simulink model "aeroblk_HL20_DG"  (Simulink 6.0)
settings: Solver=ode45  StartTime=0.0  StopTime=100  RelTol=1e-3
PreLoadFcn:
  | aeroblk_init_HL20
values from neighbouring files (symbols this model uses):
  Act2Aero = 0.5*[1 -1 0 0 0 0 0;1 1 0 0 0 0 0 ;0 0 0 0 0 0 2;0 0 1 1 0 0 0; 0 0 0 0 1 1 0;0 0 1 -1 1 -1 0;]    [aeroblk_init_HL20.m]
  Aero2Act = pinv(Act2Aero)    [aeroblk_init_HL20.m]
  Aimpoint = 12071.9115088    [aeroblk_HL20_glideslope.mat]    (also in aeroblk_init_HL20.m = 0)
  alpha0 = 0.114253174362    [aeroblk_HL20_glideslope.mat]
  hglide = [0 2.62038896415 5.2407779283 7.86116689246 10.4815558566 13.1019448208 15.7223337849 18.3427227491 20.9631117132 23.5835006774 26.2038896415 28.8242786057 ... (301 elements, 1x301)]    [aeroblk_HL20_glideslope.mat]
  qbar0 = 10722.8924586    [aeroblk_HL20_autopilot_gains.mat]
  U_trim_matrix = [-23.7683817467 -4.33440943636 4.43733647183 -22.1955716586 4.52075664841 21.6532360323 -20.4783849922 6.34956743865 19.7065472455 -22.2662158495 5.88613316784 30.8883374276 ... (120 elements, 3x8x5)]    [aeroblk_HL20_autopilot_gains.mat]
  Xglide = [0 50 100 150 200 250 300 350 400 450 500 550 ... (301 elements, 1x301)]    [aeroblk_HL20_glideslope.mat]
undefined symbols (not defined in the file or in its folder): ft, m, s
libraries: aerolibconvert x13, simulink x5, simulink3 x5, dnglibv1 x5, aeroblk_lib_HL20 x3, aerolibactuator x1
settings Model: Creator=sgage  ModifiedByFormat=rhyde  LastModifiedBy=rhyde  ModifiedComment=rhyde -- Wed Mar 13 13:42:21 2002 -- Version 1.0  ModifiedHistory=A.N.Other -- Wed Mar 13 13:42:21 2002 -- Version 1.0  ExtModeAutoUpdateStatusClock=off
settings DataIOCC: SignalLoggingName=sigsOut
settings OptimizationCC: BooleanDataType=off  InlineParams=on
settings DebuggingCC: CheckExecutionContextPreStartOutputMsg=on  CheckExecutionContextRuntimeOutputMsg=on  SolverPrmCheckMsg=none
settings HardwareCC: TargetUnknown=on
settings GRTTargetCC: LifeSpan=inf
settings SFSimCC: SFSimApplyToAllLibs=on  SFSimBuildMode=Incremental

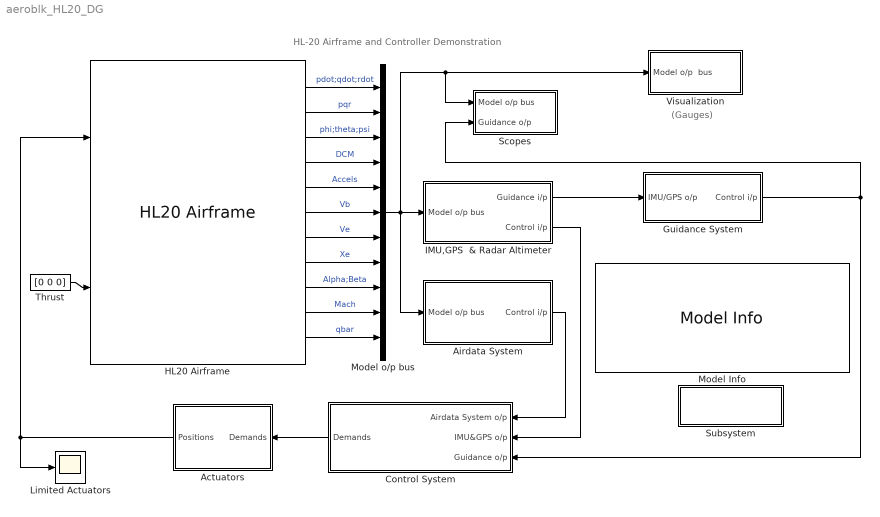
== system aeroblk_HL20_DG ==
  note: HL-20 Airframe and Controller Demonstration
  note: (Gauges)
  Actuators : Subsystem  Orientation=left  PropExecContextAcrossSSBoundary=on
  Airdata System : Subsystem  PropExecContextAcrossSSBoundary=on
  Control System : Subsystem  Orientation=left  PropExecContextAcrossSSBoundary=on
  Guidance System : Subsystem  PropExecContextAcrossSSBoundary=on
  HL20 Airframe : aeroblk_lib_HL20/HL20 Airframe
  IMU,GPS  & Radar Altimeter : Subsystem  PropExecContextAcrossSSBoundary=on
  Limited Actuators : Scope
      settings: YMin=-60  YMax=60  SaveName=ScopeData2
  Model o/p bus : BusCreator  DialogController=Simulink.DDGSource_Bus  Inputs=11
  Model Info : simulink/Model-Wide Utilities/Model Info  InitialBlockCM=None  BlockCM=None  Frame=on  DisplayStringWithTags=|  HorizontalTextAlignment=Center  LeftAlignmentValue=0.5  SourceBlockDiagram=aeroblk_HL20_DG  TagMaxNumber=20
      | HL20 version %<ModelVersion>
      | Modified on %<LastModificationDate>
      | based on 
      | Jackson E. B., Cruz C. L., 
      | "Preliminary Subsonic Aerodynamic Model for
      | Simulation Studies of the HL-20 Lifting Body", 
      | NASA TM4302, August 1992.%<Description>
  Scopes : Subsystem  PropExecContextAcrossSSBoundary=on
  Subsystem : Subsystem  PropExecContextAcrossSSBoundary=on
      settings: OpenFcn=aeroblk_lib_HL20
      mask Display: disp('Open HL20 Library')
  Thrust : Constant  Value=[0 0 0]
  Visualization : Subsystem  PropExecContextAcrossSSBoundary=on
  wires:
  Thrust/1 -> HL20 Airframe/2
  Actuators/1(Positions) -> Limited Actuators/1, HL20 Airframe/1
  Guidance System/1(Control i/p) -> Control System/3(Guidance o/p), Scopes/2(Guidance o/p)
  Control System/1(Demands) -> Actuators/1(Demands)
  HL20 Airframe/1 -> Model o/p bus/1  "pdot;qdot;rdot"
  HL20 Airframe/2 -> Model o/p bus/2  "pqr"
  HL20 Airframe/3 -> Model o/p bus/3  "phi;theta;psi"
  HL20 Airframe/4 -> Model o/p bus/4  "DCM"
  HL20 Airframe/5 -> Model o/p bus/5  "Accels"
  HL20 Airframe/6 -> Model o/p bus/6  "Vb"
  HL20 Airframe/7 -> Model o/p bus/7  "Ve"
  HL20 Airframe/8 -> Model o/p bus/8  "Xe"
  HL20 Airframe/9 -> Model o/p bus/9  "Alpha;Beta"
  HL20 Airframe/10 -> Model o/p bus/10  "Mach"
  HL20 Airframe/11 -> Model o/p bus/11  "qbar"
  Model o/p bus/1 -> Airdata System/1(Model o/p bus), IMU,GPS  & Radar Altimeter/1(Model o/p bus), Visualization/1(Model o/p  bus), Scopes/1(Model o/p bus)
  IMU,GPS  & Radar Altimeter/2(Control i/p) -> Control System/2(IMU&GPS o/p)
  Airdata System/1(Control i/p) -> Control System/1(Airdata System o/p)
  IMU,GPS  & Radar Altimeter/1(Guidance i/p) -> Guidance System/1(IMU/GPS o/p)

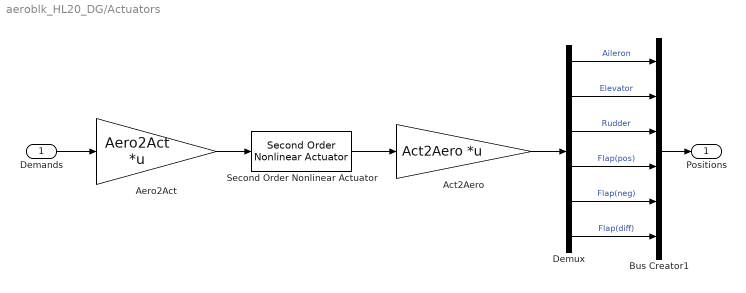
== system aeroblk_HL20_DG/Actuators ==
  Demands : Inport  LatchInput=off
  Act2Aero : Gain  Gain=Act2Aero  Multiplication=Matrix(K*u)  SaturateOnIntegerOverflow=on
  Aero2Act : Gain  Gain=Aero2Act  Multiplication=Matrix(K*u)  SaturateOnIntegerOverflow=on
  Bus Creator1 : BusCreator  DialogController=Simulink.DDGSource_Bus  Inputs=6
  Demux : Demux  Outputs=6
  Second Order Nonlinear Actuator : aerolibactuator/Second Order Nonlinear Actuator  wn_fin=wn_act  z_fin=z_act  fin_max=max_lim  fin_min=min_lim  fin_maxrate=inf  fin_act_0=0
  Positions : Outport
  wires:
  Demux/1 -> Bus Creator1/1  "Aileron"
  Demux/2 -> Bus Creator1/2  "Elevator"
  Demux/3 -> Bus Creator1/3  "Rudder"
  Demux/4 -> Bus Creator1/4  "Flap(pos)"
  Demux/5 -> Bus Creator1/5  "Flap(neg)"
  Demux/6 -> Bus Creator1/6  "Flap(diff)"
  Bus Creator1/1 -> Positions/1
  Second Order Nonlinear Actuator/1 -> Act2Aero/1
  Aero2Act/1 -> Second Order Nonlinear Actuator/1
  Act2Aero/1 -> Demux/1
  Demands/1 -> Aero2Act/1

== system aeroblk_HL20_DG/Airdata System ==
  Model o/p bus : Inport  LatchInput=off
  Bus Selector : BusSelector  DialogController=Simulink.DDGSource_Bus  OutputSignals=Alpha;Beta,qbar
  Mux : Mux  Inputs=[2,1]
  Control i/p : Outport
  wires:
  Model o/p bus/1 -> Bus Selector/1
  Bus Selector/1 -> Mux/1  "<Alpha;Beta>"
  Bus Selector/2 -> Mux/2  "<qbar>"
  Mux/1 -> Control i/p/1

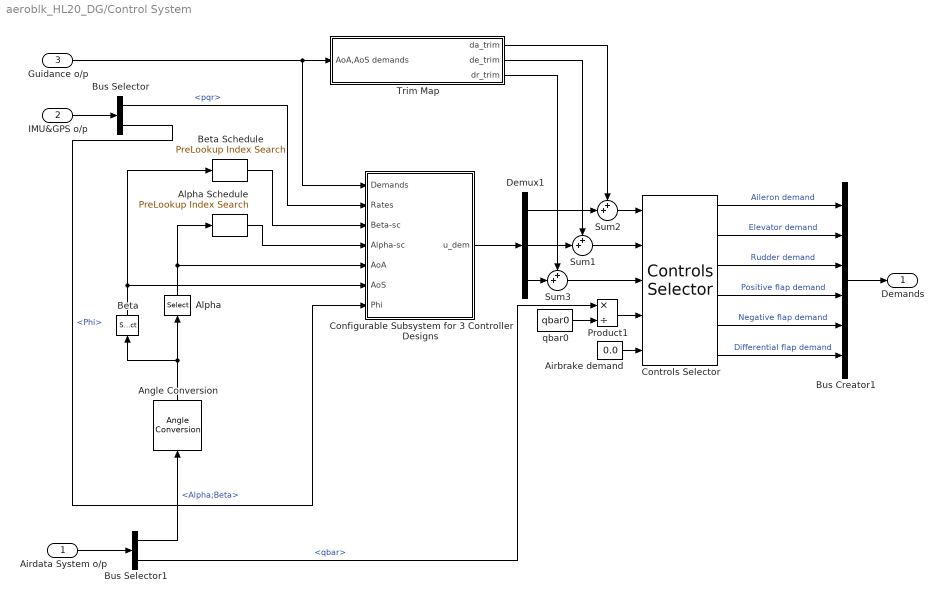
== system aeroblk_HL20_DG/Control System ==
  Airdata System o/p : Inport  LatchInput=off
  IMU&GPS o/p : Inport  Port=2  LatchInput=off
  Guidance o/p : Inport  Port=3  LatchInput=off
  Airbrake demand : Constant  Value=0.0
  Alpha : Selector  Orientation=up  InputPortWidth=2
  Alpha Schedule : simulink/Lookup Tables/PreLookup Index Search  bpData=a_vec  searchMode=Binary Search  cacheBpFlag=off  outputFlag=off  extrapMode=Linear Extrapolation  rangeErrorMode=None
  Angle Conversion : aerolibconvert/Angle Conversion  Orientation=up  IU=rad  OU=deg
  Beta : Selector  Orientation=up  Elements=2  InputPortWidth=2
  Beta Schedule : simulink/Lookup Tables/PreLookup Index Search  bpData=a_vec  searchMode=Binary Search  cacheBpFlag=off  outputFlag=off  extrapMode=Linear Extrapolation  rangeErrorMode=None
  Bus Creator1 : BusCreator  DialogController=Simulink.DDGSource_Bus  Inputs=6
  Bus Selector : BusSelector  DialogController=Simulink.DDGSource_Bus  OutputSignals=pqr,Phi
  Bus Selector1 : BusSelector  DialogController=Simulink.DDGSource_Bus  OutputSignals=Alpha;Beta,qbar
  Configurable Subsystem for 3 Controller Designs : Subsystem  BlockChoice=Classical Controller  PropExecContextAcrossSSBoundary=on
      settings: AttributesFormatString=%<BlockChoice>  MemberBlocks=Classical Controller,H-infinity Controller [1 dimensional scheduling],H-infinity Controller [2 dimensional scheduling]
      settings: TemplateBlock=|
      | aeroblk_lib_HL20/Configurable Subsystem
      | for 3 Controller Designs
  Controls Selector : aeroblk_lib_HL20/Controls Selector  SimViewingDevice=off  DataTypeOverride=UseLocalSettings  MinMaxOverflowLogging=UseLocalSettings
      settings: Permissions=ReadWrite  RTWFcnNameOpts=Auto  RTWFileNameOpts=Auto
  Demux1 : Demux  Outputs=3
  Product1 : Product  Inputs=*/  SaturateOnIntegerOverflow=on  InputSameDT=on
  Sum1 : Sum  Inputs=++|  SaturateOnIntegerOverflow=on  InputSameDT=on
  Sum2 : Sum  Inputs=++|  SaturateOnIntegerOverflow=on  InputSameDT=on
  Sum3 : Sum  Inputs=++|  SaturateOnIntegerOverflow=on  InputSameDT=on
  Trim Map : Subsystem  PropExecContextAcrossSSBoundary=on
  qbar0 : Constant  Value=qbar0
  Demands : Outport
  wires:
  Bus Creator1/1 -> Demands/1
  Alpha Schedule/1 -> Configurable Subsystem for 3 Controller Designs/4(Alpha-sc)
  Beta Schedule/1 -> Configurable Subsystem for 3 Controller Designs/3(Beta-sc)
  Bus Selector/1 -> Configurable Subsystem for 3 Controller Designs/2(Rates)  "<pqr>"
  Guidance o/p/1 -> Trim Map/1(AoA,AoS demands), Configurable Subsystem for 3 Controller Designs/1(Demands)
  Alpha/1 -> Alpha Schedule/1, Configurable Subsystem for 3 Controller Designs/5(AoA)
  Angle Conversion/1 -> Beta/1, Alpha/1
  Controls Selector/1 -> Bus Creator1/1  "Aileron demand"
  Controls Selector/2 -> Bus Creator1/2  "Elevator demand"
  Controls Selector/3 -> Bus Creator1/3  "Rudder demand"
  Controls Selector/4 -> Bus Creator1/4  "Positive flap demand"
  Controls Selector/5 -> Bus Creator1/5  "Negative flap demand"
  Controls Selector/6 -> Bus Creator1/6  "Differential flap demand"
  Beta/1 -> Beta Schedule/1, Configurable Subsystem for 3 Controller Designs/6(AoS)
  Product1/1 -> Controls Selector/4
  qbar0/1 -> Product1/2
  Sum2/1 -> Controls Selector/1
  Trim Map/1(da_trim) -> Sum2/1
  Sum1/1 -> Controls Selector/2
  Sum3/1 -> Controls Selector/3
  Trim Map/2(de_trim) -> Sum1/1
  Trim Map/3(dr_trim) -> Sum3/1
  Demux1/2 -> Sum1/2
  Demux1/3 -> Sum3/2
  Demux1/1 -> Sum2/2
  Configurable Subsystem for 3 Controller Designs/1(u_dem) -> Demux1/1
  IMU&GPS o/p/1 -> Bus Selector/1
  Bus Selector/2 -> Configurable Subsystem for 3 Controller Designs/7(Phi)  "<Phi>"
  Airdata System o/p/1 -> Bus Selector1/1
  Bus Selector1/1 -> Angle Conversion/1  "<Alpha;Beta>"
  Bus Selector1/2 -> Product1/1  "<qbar>"
  Airbrake demand/1 -> Controls Selector/5

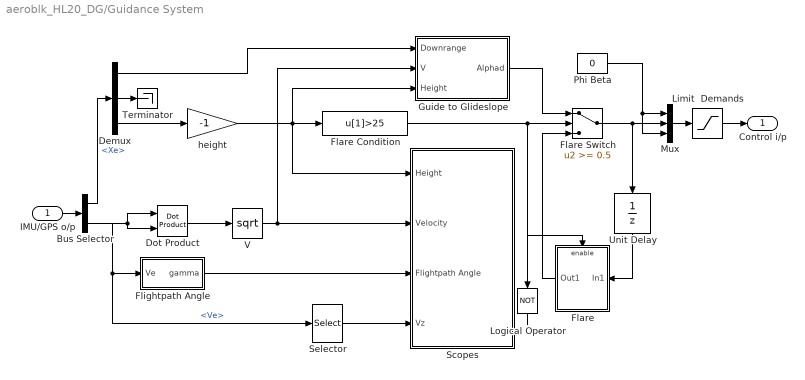
== system aeroblk_HL20_DG/Guidance System ==
  IMU/GPS o/p : Inport  LatchInput=off
  Bus Selector : BusSelector  DialogController=Simulink.DDGSource_Bus  OutputSignals=Xe,Ve
  Demux : Demux  Outputs=3
  Dot Product : simulink/Math Operations/Dot Product  OutDataType=sfix(16)  OutScaling=2^-10  DoSatur=on
  Flare : Subsystem  Orientation=left  TreatAsAtomicUnit=on  PropExecContextAcrossSSBoundary=on
  Flare Condition : Fcn  Expr=u[1]>25
  Flare Switch : Switch  Threshold=0.5  SaturateOnIntegerOverflow=on  InputSameDT=on
  Flightpath Angle : Subsystem  PropExecContextAcrossSSBoundary=on
  Guide to Glideslope : Subsystem  PropExecContextAcrossSSBoundary=on
  Limit  Demands : Saturate  UpperLimit=[20 25 5]  LowerLimit=[-20 -10 -5]
  Logical Operator : Logic  Orientation=down  Operator=NOT
  Mux : Mux  Inputs=3
  Phi Beta : Constant  Value=0
  Scopes : Subsystem  PropExecContextAcrossSSBoundary=on
  Selector : Selector  Elements=[3]  InputPortWidth=3
  Terminator : Terminator
  Unit Delay : UnitDelay  Orientation=down  SampleTime=0.1
  V : Math  Operator=sqrt  SaturateOnIntegerOverflow=on
  height : Gain  Gain=-1  SaturateOnIntegerOverflow=on
  Control i/p : Outport
  wires:
  Dot Product/1 -> V/1
  Unit Delay/1 -> Flare/1(In1)
  Logical Operator/1 -> Flare/Enable
  Demux/2 -> Terminator/1
  Guide to Glideslope/1(Alphad) -> Flare Switch/1
  Limit  Demands/1 -> Control i/p/1
  Flare/1(Out1) -> Flare Switch/3
  Flare Switch/1 -> Unit Delay/1, Mux/2
  Flare Condition/1 -> Logical Operator/1, Flare Switch/2
  Phi Beta/1 -> Mux/1, Mux/3
  Selector/1 -> Scopes/4(Vz)
  V/1 -> Scopes/2(Velocity), Guide to Glideslope/2(V)
  Mux/1 -> Limit  Demands/1
  height/1 -> Scopes/1(Height), Guide to Glideslope/3(Height), Flare Condition/1
  Demux/3 -> height/1
  Demux/1 -> Guide to Glideslope/1(Downrange)
  Bus Selector/1 -> Demux/1  "<Xe>"
  Flightpath Angle/1(gamma) -> Scopes/3(Flightpath Angle)
  Bus Selector/2 -> Flightpath Angle/1(Ve), Dot Product/2, Dot Product/1, Selector/1  "<Ve>"
  IMU/GPS o/p/1 -> Bus Selector/1

== system aeroblk_HL20_DG/IMU,GPS  & Radar Altimeter ==
  Model o/p bus : Inport  LatchInput=off
  Bus Creator : BusCreator  DialogController=Simulink.DDGSource_Bus  Inputs=7
  Bus Selector : BusSelector  DialogController=Simulink.DDGSource_Bus  OutputSignals=pqr,phi;theta;psi,DCM,Accels,Vb,Ve,Xe
  Mux : Mux  Inputs=[3,1]
  Select Phi : Selector  Elements=[1]  InputPortWidth=3
  Guidance i/p : Outport
  Control i/p : Outport  Port=2
  wires:
  Model o/p bus/1 -> Bus Selector/1
  Bus Selector/1 -> Bus Creator/1, Mux/1  "<pqr>"
  Bus Selector/2 -> Bus Creator/2, Select Phi/1  "<phi;theta;psi>"
  Bus Selector/3 -> Bus Creator/3  "<DCM>"
  Bus Selector/4 -> Bus Creator/4  "<Accels>"
  Bus Selector/5 -> Bus Creator/5  "<Vb>"
  Bus Selector/6 -> Bus Creator/6  "<Ve>"
  Bus Selector/7 -> Bus Creator/7  "<Xe>"
  Bus Creator/1 -> Guidance i/p/1
  Select Phi/1 -> Mux/2  "Phi"
  Mux/1 -> Control i/p/1

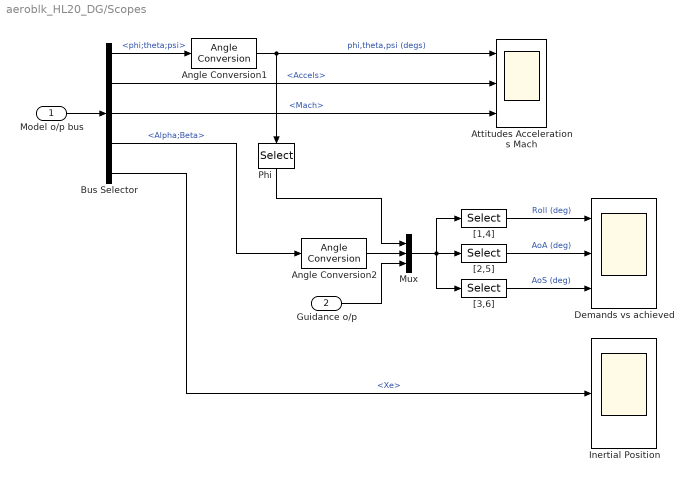
== system aeroblk_HL20_DG/Scopes ==
  Model o/p bus : Inport  LatchInput=off
  Guidance o/p : Inport  Port=2  LatchInput=off
  Angle Conversion1 : aerolibconvert/Angle Conversion  IU=rad  OU=deg
  Angle Conversion2 : aerolibconvert/Angle Conversion  IU=rad  OU=deg
  Attitudes Accelerations Mach : Scope  NumInputPorts=3
      settings: YMin=-11~-1.25~0.581  YMax=1~1.75~0.595  SaveName=ScopeData3  Decimation=5
  Bus Selector : BusSelector  DialogController=Simulink.DDGSource_Bus  OutputSignals=phi;theta;psi,Accels,Mach,Alpha;Beta,Xe
  Demands vs achieved : Scope  NumInputPorts=3
      settings: TimeRange=100  YMin=-0.6~2.5~-0.7  YMax=0.7~22.5~0.6  Decimation=5
  Inertial Position : Scope
      settings: TimeRange=100  YMin=-13000  YMax=1000  Decimation=5
  Mux : Mux  Inputs=[1,2,3]
  Phi : Selector  Orientation=down  InputPortWidth=3
  "[1,4]" : Selector  Elements=[1 4]  InputPortWidth=6
  "[2,5]" : Selector  Elements=[2 5]  InputPortWidth=6
  "[3,6]" : Selector  Elements=[3 6]  InputPortWidth=6
  wires:
  Model o/p bus/1 -> Bus Selector/1
  Bus Selector/1 -> Angle Conversion1/1  "<phi;theta;psi>"
  Bus Selector/2 -> Attitudes Accelerations Mach/2  "<Accels>"
  Bus Selector/3 -> Attitudes Accelerations Mach/3  "<Mach>"
  Phi/1 -> Mux/1
  Bus Selector/4 -> Angle Conversion2/1  "<Alpha;Beta>"
  Angle Conversion2/1 -> Mux/2
  Mux/1 -> "[1,4]"/1, "[2,5]"/1, "[3,6]"/1
  Guidance o/p/1 -> Mux/3
  "[1,4]"/1 -> Demands vs achieved/1  "Roll (deg)"
  "[2,5]"/1 -> Demands vs achieved/2  "AoA (deg)"
  "[3,6]"/1 -> Demands vs achieved/3  "AoS (deg)"
  Bus Selector/5 -> Inertial Position/1  "<Xe>"
  Angle Conversion1/1 -> Phi/1, Attitudes Accelerations Mach/1  "phi,theta,psi (degs)"

== system aeroblk_HL20_DG/Subsystem ==

== system aeroblk_HL20_DG/Visualization ==
  Model o/p  bus : Inport  LatchInput=off
  AirSpeed : dnglibv1/ActiveX Control  progid=air.airctrl.1  connect=input  input=airspeed  init=hActx.displaymode=4;  inblock=on  border=off  dialOut=0  updateParam=0
  Altimeter : dnglibv1/ActiveX Control  progid=air.airctrl.1  connect=input  input=altitude  init=hActx.displaymode=2;hActx.altthousandstyle=1;  inblock=on  border=off  dialOut=0  updateParam=0
  Artificial Horizon : dnglibv1/ActiveX Control  progid=air.airctrl.1  connect=input  input=ahroll, ahpitch  init=hActx.displaymode=6;  inblock=on  border=off  dialOut=0  updateParam=0
  Climb Rate : dnglibv1/ActiveX Control  progid=air.airctrl.1  connect=input  input=climbrate  init=hActx.displaymode=3;  inblock=on  border=off  dialOut=0  updateParam=0
  Extract Gauges : Subsystem  PropExecContextAcrossSSBoundary=on
  Heading Indicator : dnglibv1/ActiveX Control  progid=air.airctrl.1  connect=input  init=hActx.displaymode=1;  inblock=on  border=off  dialOut=0  updateParam=0
  wires:
  Model o/p  bus/1 -> Extract Gauges/1(Demands)
  Extract Gauges/1(Airspeed (kts)) -> AirSpeed/1
  Extract Gauges/5(Heading (deg)) -> Heading Indicator/1
  Extract Gauges/2(Height (ft)) -> Altimeter/1
  Extract Gauges/4(Climb Rate (ft/min)) -> Climb Rate/1
  Extract Gauges/3(Roll Flightpath (deg)) -> Artificial Horizon/1

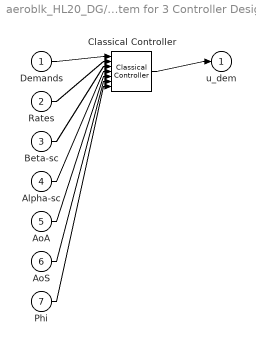
== system aeroblk_HL20_DG/Control System/Configurable Subsystem for 3 Controller Designs ==
  Demands : Inport  LatchInput=off
  Rates : Inport  Port=2  LatchInput=off
  Beta-sc : Inport  Port=3  LatchInput=off
  Alpha-sc : Inport  Port=4  LatchInput=off
  AoA : Inport  Port=5  LatchInput=off
  AoS : Inport  Port=6  LatchInput=off
  Phi : Inport  Port=7  LatchInput=off
  Classical Controller : aeroblk_lib_HL20/Classical Controller  SimViewingDevice=off  DataTypeOverride=UseLocalSettings  MinMaxOverflowLogging=UseLocalSettings
      settings: Permissions=ReadWrite  RTWFcnNameOpts=Auto  RTWFileNameOpts=Auto
  u_dem : Outport
  wires:
  Demands/1 -> Classical Controller/1
  Rates/1 -> Classical Controller/2
  Beta-sc/1 -> Classical Controller/3
  Alpha-sc/1 -> Classical Controller/4
  AoA/1 -> Classical Controller/5
  AoS/1 -> Classical Controller/6
  Phi/1 -> Classical Controller/7
  Classical Controller/1 -> u_dem/1

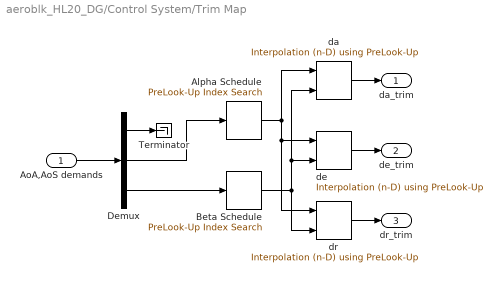
== system aeroblk_HL20_DG/Control System/Trim Map ==
  AoA,AoS demands : Inport  LatchInput=off
  Alpha Schedule : simulink3/Functions & Tables/PreLook-Up Index Search  bpData=a_vec  searchMode=Binary Search  cacheBpFlag=on  outputFlag=off  extrapMode=Linear Extrapolation  rangeErrorMode=None
  Beta Schedule : simulink3/Functions & Tables/PreLook-Up Index Search  bpData=a_vec  searchMode=Binary Search  cacheBpFlag=on  outputFlag=off  extrapMode=Linear Extrapolation  rangeErrorMode=None
  Demux : Demux  Outputs=3
  Terminator : Terminator
  da : simulink3/Functions & Tables/Interpolation (n-D) using PreLook-Up  numDimsPopupSelect=2  explicitNumDims=2  table=squeeze(U_trim_matrix(1,:,:))  interpMethod=Linear  extrapMethod=Linear  rangeErrorMode=None
  de : simulink3/Functions & Tables/Interpolation (n-D) using PreLook-Up  numDimsPopupSelect=2  explicitNumDims=2  table=squeeze(U_trim_matrix(2,:,:))  interpMethod=Linear  extrapMethod=Linear  rangeErrorMode=None
  dr : simulink3/Functions & Tables/Interpolation (n-D) using PreLook-Up  numDimsPopupSelect=2  explicitNumDims=2  table=squeeze(U_trim_matrix(3,:,:))  interpMethod=Linear  extrapMethod=Linear  rangeErrorMode=None
  da_trim : Outport
  de_trim : Outport  Port=2
  dr_trim : Outport  Port=3
  wires:
  Alpha Schedule/1 -> da/1, de/1, dr/1
  Beta Schedule/1 -> da/2, de/2, dr/2
  AoA,AoS demands/1 -> Demux/1
  Demux/2 -> Alpha Schedule/1
  Demux/3 -> Beta Schedule/1
  Demux/1 -> Terminator/1
  da/1 -> da_trim/1
  de/1 -> de_trim/1
  dr/1 -> dr_trim/1

== system aeroblk_HL20_DG/Guidance System/Flare ==
  In1 : Inport  LatchInput=off
  Enable : EnablePort  StatesWhenEnabling=reset
  Alphad1 : Integrator  InitialConditionSource=external
  Flare Demand1 : Constant  Value=17.5
  Gain1 : Gain  Gain=2  SaturateOnIntegerOverflow=on
  Sum2 : Sum  Inputs=|+-  SaturateOnIntegerOverflow=on  InputSameDT=on
  Out1 : Outport  InitialOutput=[0]
  wires:
  Alphad1/1 -> Out1/1, Sum2/2
  Gain1/1 -> Alphad1/1
  Sum2/1 -> Gain1/1
  Flare Demand1/1 -> Sum2/1
  In1/1 -> Alphad1/2

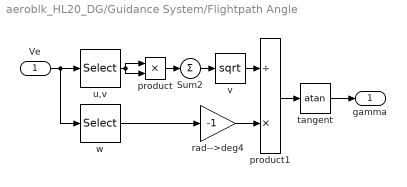
== system aeroblk_HL20_DG/Guidance System/Flightpath Angle ==
  Ve : Inport  LatchInput=off
  Sum2 : Sum  Inputs=+  SaturateOnIntegerOverflow=on  InputSameDT=on
  product : Product  SaturateOnIntegerOverflow=on  InputSameDT=on
  product1 : Product  Inputs=/*  SaturateOnIntegerOverflow=on  InputSameDT=on
  rad-->deg4 : Gain  Gain=-1  SaturateOnIntegerOverflow=on
  tangent : Trigonometry  Operator=atan
  u,v : Selector  Elements=[1 2]  InputPortWidth=3
  v : Math  Operator=sqrt  SaturateOnIntegerOverflow=on
  w : Selector  Elements=3  InputPortWidth=3
  gamma : Outport
  wires:
  w/1 -> rad-->deg4/1
  u,v/1 -> product/1, product/2
  v/1 -> product1/1
  rad-->deg4/1 -> product1/2
  product1/1 -> tangent/1
  Sum2/1 -> v/1
  product/1 -> Sum2/1
  Ve/1 -> u,v/1, w/1
  tangent/1 -> gamma/1

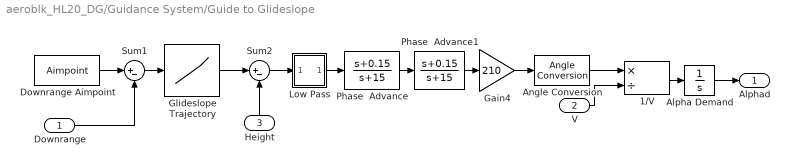
== system aeroblk_HL20_DG/Guidance System/Guide to Glideslope ==
  Downrange : Inport  LatchInput=off
  V : Inport  Port=2  LatchInput=off
  Height : Inport  Orientation=up  Port=3  LatchInput=off
  1/V : Product  Inputs=*/  SaturateOnIntegerOverflow=on  InputSameDT=on
  Alpha Demand : Integrator  InitialCondition=alpha0*180/pi
  Angle Conversion : aerolibconvert/Angle Conversion  IU=rad  OU=deg
  Downrange Aimpoint : Constant  Value=Aimpoint
  Gain4 : Gain  Gain=210  SaturateOnIntegerOverflow=on
  Glideslope Trajectory : Lookup  DialogController=Simulink.DDGSource  InputValues=Xglide  OutputValues=hglide  SaturateOnIntegerOverflow=on
  Low Pass : Subsystem  PropExecContextAcrossSSBoundary=on
  Phase  Advance : TransferFcn  Numerator=[1 0.15]  Denominator=[1 15]
  Phase  Advance1 : TransferFcn  Numerator=[1 0.15]  Denominator=[1 15]
  Sum1 : Sum  Inputs=|+-  SaturateOnIntegerOverflow=on  InputSameDT=on
  Sum2 : Sum  Inputs=|+-  SaturateOnIntegerOverflow=on  InputSameDT=on
  Alphad : Outport
  wires:
  Angle Conversion/1 -> 1/V/1
  Downrange/1 -> Sum1/2
  Alpha Demand/1 -> Alphad/1
  Height/1 -> Sum2/2
  V/1 -> 1/V/2
  Low Pass/1(Out1) -> Phase  Advance/1
  1/V/1 -> Alpha Demand/1
  Gain4/1 -> Angle Conversion/1
  Phase  Advance/1 -> Phase  Advance1/1
  Phase  Advance1/1 -> Gain4/1
  Sum2/1 -> Low Pass/1(In1)
  Glideslope Trajectory/1 -> Sum2/1
  Sum1/1 -> Glideslope Trajectory/1
  Downrange Aimpoint/1 -> Sum1/1

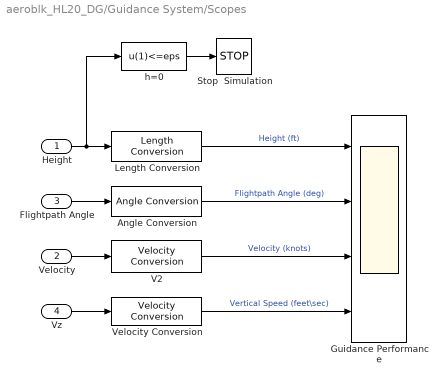
== system aeroblk_HL20_DG/Guidance System/Scopes ==
  Height : Inport  LatchInput=off
  Velocity : Inport  Port=2  LatchInput=off
  Flightpath Angle : Inport  Port=3  LatchInput=off
  Vz : Inport  Port=4  LatchInput=off
  Angle Conversion : aerolibconvert/Angle Conversion  IU=rad  OU=deg
  Guidance Performance : Scope  NumInputPorts=4
      settings: TimeRange=70  YMin=0~-20~200~0  YMax=10000~0~400~225  SaveName=ScopeData6
  Length Conversion : aerolibconvert/Length Conversion  IU=m  OU=ft
  Stop  Simulation : Stop
  V2 : aerolibconvert/Velocity Conversion  IU=m/s  OU=kts
  Velocity Conversion : aerolibconvert/Velocity Conversion  IU=m/s  OU=ft/s
  h=0 : Fcn  Expr=u(1)<=eps
  wires:
  h=0/1 -> Stop  Simulation/1
  Vz/1 -> Velocity Conversion/1
  Flightpath Angle/1 -> Angle Conversion/1
  Height/1 -> h=0/1, Length Conversion/1
  Velocity/1 -> V2/1
  Length Conversion/1 -> Guidance Performance/1  "Height (ft)"
  V2/1 -> Guidance Performance/3  "Velocity (knots)"
  Velocity Conversion/1 -> Guidance Performance/4  "Vertical Speed (feet\\sec)"
  Angle Conversion/1 -> Guidance Performance/2  "Flightpath Angle (deg)"

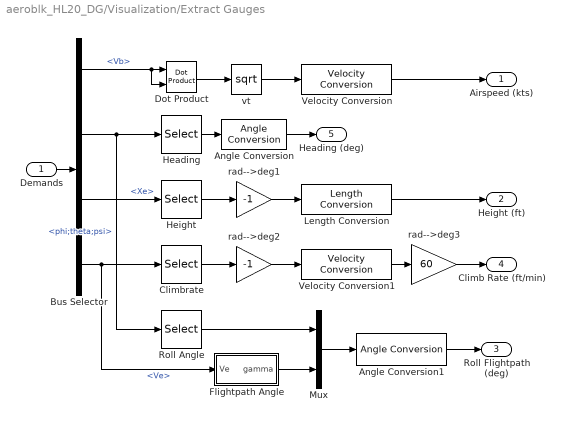
== system aeroblk_HL20_DG/Visualization/Extract Gauges ==
  Demands : Inport  LatchInput=off
  Angle Conversion : aerolibconvert/Angle Conversion  IU=rad  OU=deg
  Angle Conversion1 : aerolibconvert/Angle Conversion  IU=rad  OU=deg
  Bus Selector : BusSelector  DialogController=Simulink.DDGSource_Bus  OutputSignals=Vb,phi;theta;psi,Xe,Ve
  Climbrate : Selector  Elements=[3]  InputPortWidth=3
  Dot Product : simulink/Math Operations/Dot Product  OutDataType=sfix(16)  OutScaling=2^-10  DoSatur=on
  Flightpath Angle : Subsystem  PropExecContextAcrossSSBoundary=on
  Heading : Selector  Elements=[3]  InputPortWidth=3
  Height : Selector  Elements=[3]  InputPortWidth=3
  Length Conversion : aerolibconvert/Length Conversion  IU=m  OU=ft
  Mux : Mux  Inputs=2
  Roll Angle : Selector  Elements=[1]  InputPortWidth=3
  Velocity Conversion : aerolibconvert/Velocity Conversion  IU=m/s  OU=kts
  Velocity Conversion1 : aerolibconvert/Velocity Conversion  IU=m/s  OU=ft/s
  rad-->deg1 : Gain  Gain=-1  SaturateOnIntegerOverflow=on
  rad-->deg2 : Gain  Gain=-1  SaturateOnIntegerOverflow=on
  rad-->deg3 : Gain  Gain=60  SaturateOnIntegerOverflow=on
  vt : Math  Operator=sqrt  SaturateOnIntegerOverflow=on
  Airspeed (kts) : Outport
  Height (ft) : Outport  Port=2
  Roll Flightpath (deg) : Outport  Port=3
  Climb Rate (ft/min) : Outport  Port=4
  Heading (deg) : Outport  Port=5
  wires:
  Flightpath Angle/1(gamma) -> Mux/2
  Angle Conversion1/1 -> Roll Flightpath (deg)/1
  Mux/1 -> Angle Conversion1/1
  Roll Angle/1 -> Mux/1
  rad-->deg3/1 -> Climb Rate (ft/min)/1
  Velocity Conversion1/1 -> rad-->deg3/1
  Bus Selector/4 -> Flightpath Angle/1(Ve), Climbrate/1  "<Ve>"
  rad-->deg2/1 -> Velocity Conversion1/1
  Climbrate/1 -> rad-->deg2/1
  Length Conversion/1 -> Height (ft)/1
  rad-->deg1/1 -> Length Conversion/1
  Height/1 -> rad-->deg1/1
  Bus Selector/3 -> Height/1  "<Xe>"
  Angle Conversion/1 -> Heading (deg)/1
  Heading/1 -> Angle Conversion/1
  Bus Selector/2 -> Roll Angle/1, Heading/1  "<phi;theta;psi>"
  Velocity Conversion/1 -> Airspeed (kts)/1
  vt/1 -> Velocity Conversion/1
  Dot Product/1 -> vt/1
  Bus Selector/1 -> Dot Product/2, Dot Product/1  "<Vb>"
  Demands/1 -> Bus Selector/1

== system aeroblk_HL20_DG/Guidance System/Guide to Glideslope/Low Pass ==
  In1 : Inport  LatchInput=off
  Integrator : Integrator  InitialConditionSource=external
  Omega : Gain  Gain=2  SaturateOnIntegerOverflow=on
  Sum3 : Sum  Inputs=|+-  SaturateOnIntegerOverflow=on  InputSameDT=on
  Out1 : Outport
  wires:
  In1/1 -> Integrator/2, Sum3/1
  Integrator/1 -> Out1/1, Sum3/2
  Sum3/1 -> Omega/1
  Omega/1 -> Integrator/1

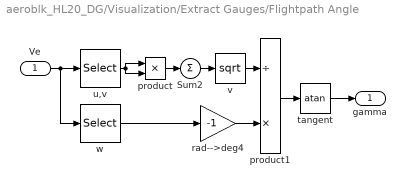
== system aeroblk_HL20_DG/Visualization/Extract Gauges/Flightpath Angle ==
  Ve : Inport  LatchInput=off
  Sum2 : Sum  Inputs=+  SaturateOnIntegerOverflow=on  InputSameDT=on
  product : Product  SaturateOnIntegerOverflow=on  InputSameDT=on
  product1 : Product  Inputs=/*  SaturateOnIntegerOverflow=on  InputSameDT=on
  rad-->deg4 : Gain  Gain=-1  SaturateOnIntegerOverflow=on
  tangent : Trigonometry  Operator=atan
  u,v : Selector  Elements=[1 2]  InputPortWidth=3
  v : Math  Operator=sqrt  SaturateOnIntegerOverflow=on
  w : Selector  Elements=3  InputPortWidth=3
  gamma : Outport
  wires:
  tangent/1 -> gamma/1
  Ve/1 -> w/1, u,v/1
  product/1 -> Sum2/1
  Sum2/1 -> v/1
  product1/1 -> tangent/1
  rad-->deg4/1 -> product1/2
  v/1 -> product1/1
  u,v/1 -> product/2, product/1
  w/1 -> rad-->deg4/1
